simulink model "CR"  (R2020a)
settings: Solver=FixedStepAuto  StartTime=0.0  StopTime=0.02  FixedStep=1e-6  RelTol=1e-3
values from neighbouring files (symbols this model uses):
  A = 50    [injecktion.m]
  A_cyl = (pi*i_n/4)*d_noz^2    (= 4.31247208956e-07)    [injecktion.m]
  A_i = pi/4*d_i^2    (= 8.04247719319e-06)    [injecktion.m]
  A_n = (pi/4)*d_n^2    (= 6.93977817178e-05)    [injecktion.m]
  A_p = (pi/4)*d_p^2    (= 6.93977817178e-05)    [injecktion.m]
  A_pis = (pi/4)*d_p^2    (= 6.93977817178e-05)    [injecktion.m]
  A_s = (pi/4)*d_s^2    (= 3.63168110755e-05)    [injecktion.m]
  A_v = (pi/4)*d_c^2    (= 8.04247719319e-06)    [injecktion.m]
  angl = kamaz{1:720,1} - 180    [injecktion.m]
  angl_inj = [150 166.5 166.6 169.4 169.5 180.2 180.3 200]    [injecktion.m]
  B = -20    [injecktion.m]
  b_b = 0.2    [injecktion.m]
  b_n = 0.3    [injecktion.m]
  C_di = 0.85    [injecktion.m]
  Hv_max = 0.00052    [injecktion.m]
  K_n = 270000    [injecktion.m]
  K_v = 220000    [injecktion.m]
  L = 0.0002    [injecktion.m]
  m_a = 0.020    (= 0.02)    [injecktion.m]
  m_sum = 0.032    [injecktion.m]
  P_cyl = kamaz{1:720,2}    [injecktion.m]
  P_rail = 1800    [injecktion.m]
  P_t = 5    [injecktion.m]
  R = 1.1    [injecktion.m]
  rho = 832    [injecktion.m]
  V_inj = [0 0 60 60 40 40 0 0]    [injecktion.m]
libraries: simulink x1
settings Model: Creator=manun  LastModifiedBy=manun
settings SolverCC: AlgebraicLoopSolver=LineSearch

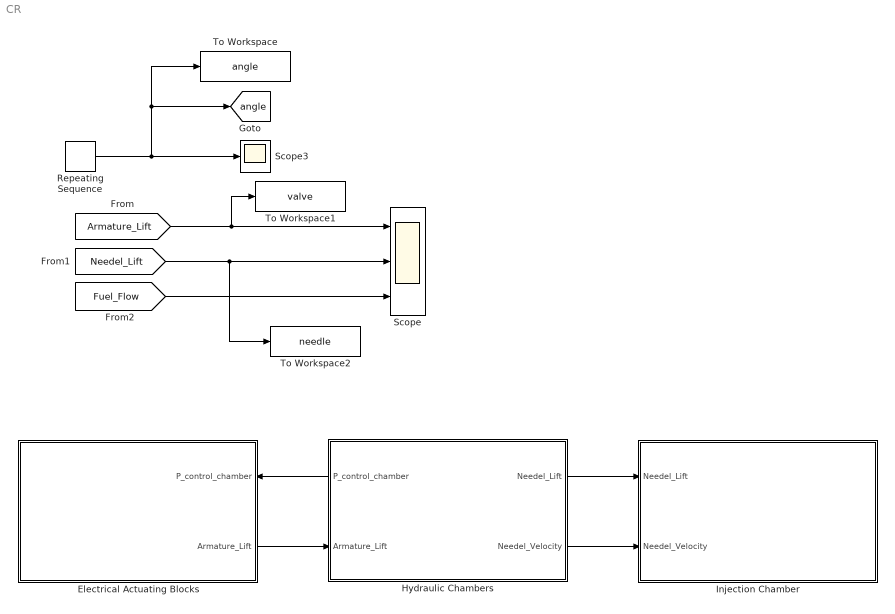
== system CR ==
  Electrical Actuating Blocks : Subsystem
      settings: PortSchema="{\"entries\":[{\"content\":{\"sides\":[{\"content\":{\"connectorIds\":[]},\"type\":\"ConnectorPlacement.EquallySpacedRectSide\",\"uuid\":\"3ba77c4c-b8ba-4d77-9d68-8710a2d773ab\"},{\"content\":{\"connectorIds\":[\"In1\",\"Out1\"],\"side\":\"RIGHT\"},\"type\":\"ConnectorPlacement.EquallySpacedRectSide\",\"uuid\":\"fd57f4f6-7259-4663-815b-091bcd4e1737\"},{\"content\":{\"connectorIds\":[],\"side\":\"TOP\"},\"type\":\"ConnectorPlacement.EquallySpacedRectSide\",\"uuid\":\"95c5c282-81a4-45f7-9203-cb060914cd9c\"}]},\"type\":\"ConnectorPlacement.EquallySpacedConnector\",\"uuid\":\"804a231b-9b03-46bc-815b-f5b483ae5845\"}],\"packageUris\":[\"http://schema.mathworks.com/mf0/Connector/19700101\"],\"version\":\"1.0\"}"
  Hydraulic Chambers : Subsystem
      settings: PortSchema="{\"entries\":[{\"content\":{\"sides\":[{\"content\":{\"connectorIds\":[\"Out3\",\"In1\"]},\"type\":\"ConnectorPlacement.EquallySpacedRectSide\",\"uuid\":\"e260e5f4-acfe-4da7-b401-bae8e315cc37\"},{\"content\":{\"connectorIds\":[\"Out1\",\"Out2\"],\"side\":\"RIGHT\"},\"type\":\"ConnectorPlacement.EquallySpacedRectSide\",\"uuid\":\"01019c56-b8d4-4519-8d57-ed1d2bc069d1\"},{\"content\":{\"connectorIds\":[],\"side\":\"TOP\"},\"type\":\"ConnectorPlacement.EquallySpacedRectSide\",\"uuid\":\"98af096b-7f3f-48cd-9514-e14eeceb55ee\"}]},\"type\":\"ConnectorPlacement.EquallySpacedConnector\",\"uuid\":\"efa95c2f-1e5f-488c-845f-cfa36b8d7348\"}],\"packageUris\":[\"http://schema.mathworks.com/mf0/Connector/19700101\"],\"version\":\"1.0\"}"
  Injection Chamber : Subsystem
  Repeating Sequence : simulink/Sources/Repeating Sequence  rep_seq_t=[0 0.0632]  rep_seq_y=[0 720]
  Scope : Scope  NumInputPorts=3
  Scope3 : Scope
  To Workspace : ToWorkspace  VariableName=angle  SampleTime=-1
  To Workspace1 : ToWorkspace  VariableName=valve  SaveFormat=Timeseries  SampleTime=-1
  To Workspace2 : ToWorkspace  VariableName=needle  SaveFormat=Timeseries  SampleTime=-1
  tag scope: angle=global
  wires:
  Repeating Sequence/1 -> To Workspace/1, [angle], Scope3/1
  Electrical Actuating Blocks/1(Armature_Lift) -> Hydraulic Chambers/1(Armature_Lift)
  Hydraulic Chambers/3(P_control_chamber) -> Electrical Actuating Blocks/1(P_control_chamber)
  Hydraulic Chambers/1(Needel_Lift) -> Injection Chamber/1(Needel_Lift)
  Hydraulic Chambers/2(Needel_Velocity) -> Injection Chamber/2(Needel_Velocity)
  [Armature_Lift] -> To Workspace1/1, Scope/1
  [Needel_Lift] -> To Workspace2/1, Scope/2
  [Fuel_Flow] -> Scope/3

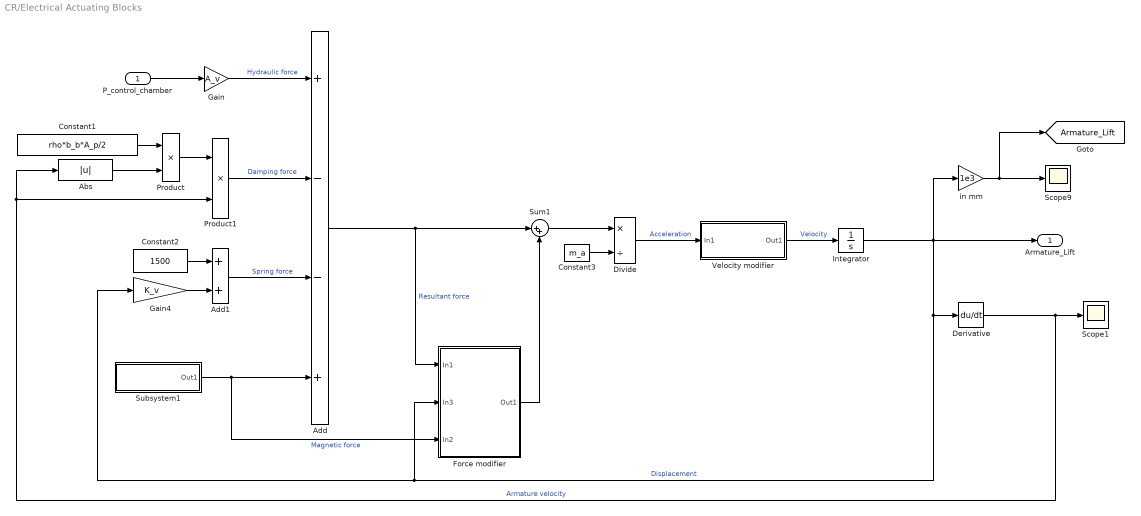
== system CR/Electrical Actuating Blocks ==
  P_control_chamber : Inport
  Abs : Abs
  Add : Sum  Inputs=+--+
  Add1 : Sum
  Constant1 : Constant  Value=rho*b_b*A_p/2
  Constant2 : Constant  Value=1500
  Constant3 : Constant  Value=m_a
  Derivative : Derivative
  Divide : Product  Inputs=*/
  Force modifier : Subsystem
  Gain : Gain  Gain=A_v
  Gain4 : Gain  Gain=K_v
  Integrator : Integrator  LimitOutput=on  UpperSaturationLimit=Hv_max  LowerSaturationLimit=0
  Product : Product
  Product1 : Product
  Scope1 : Scope
  Scope9 : Scope
  Subsystem1 : Subsystem
  Sum1 : Sum  Inputs=|++
  Velocity modifier : Subsystem
  in mm : Gain  Gain=1e3
  Armature_Lift : Outport
  tag scope: Armature_Lift=global
  wires:
  Integrator/1 -> Force modifier/2(In3), Gain4/1, Derivative/1, Armature_Lift/1, in mm/1  "Displacement"
  Constant3/1 -> Divide/2
  Gain4/1 -> Add1/2
  Sum1/1 -> Divide/1
  Add/1 -> Force modifier/1(In1), Sum1/1  "Resultant force"
  Abs/1 -> Product/2
  Velocity modifier/1(Out1) -> Integrator/1  "Velocity"
  P_control_chamber/1 -> Gain/1
  Product1/1 -> Add/2  "Damping force"
  Force modifier/1(Out1) -> Sum1/2
  Derivative/1 -> Scope1/1, Product1/2, Abs/1  "Armature velocity"
  Divide/1 -> Velocity modifier/1(In1)  "Acceleration"
  Product/1 -> Product1/1
  Constant2/1 -> Add1/1
  Subsystem1/1(Out1) -> Force modifier/3(In2), Add/4  "Magnetic force"
  Gain/1 -> Add/1  "Hydraulic force"
  Constant1/1 -> Product/1
  in mm/1 -> [Armature_Lift], Scope9/1
  Add1/1 -> Add/3  "Spring force"

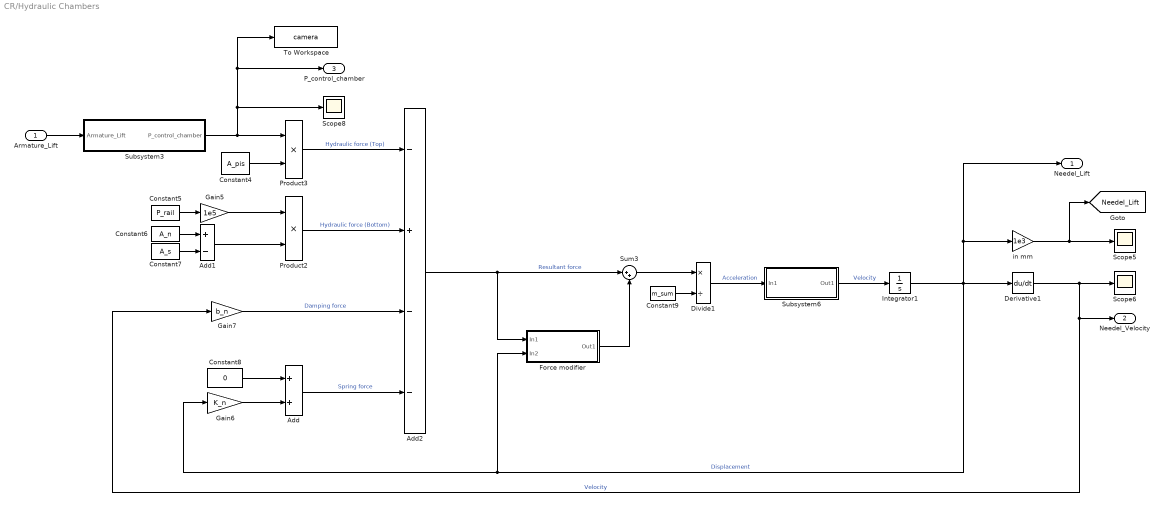
== system CR/Hydraulic Chambers ==
  Armature_Lift : Inport
  Add : Sum
  Add1 : Sum  Inputs=+-
  Add2 : Sum  Inputs=-+--
  Constant4 : Constant  Value=A_pis
  Constant5 : Constant  Value=P_rail
  Constant6 : Constant  Value=A_n
  Constant7 : Constant  Value=A_s
  Constant8 : Constant  Value=0
  Constant9 : Constant  Value=m_sum
  Derivative1 : Derivative
  Divide1 : Product  Inputs=*/
  Force modifier : Subsystem
  Gain5 : Gain  Gain=1e5
  Gain6 : Gain  Gain=K_n
  Gain7 : Gain  Gain=b_n
  Integrator1 : Integrator  LimitOutput=on  LowerSaturationLimit=0
  Product2 : Product
  Product3 : Product
  Scope5 : Scope
  Scope6 : Scope
  Scope8 : Scope
  Subsystem3 : Subsystem
  Subsystem6 : Subsystem
  Sum3 : Sum  Inputs=|++
  To Workspace : ToWorkspace  VariableName=camera  SaveFormat=Timeseries  SampleTime=-1
  in mm : Gain  Gain=1e3
  Needel_Lift : Outport
  Needel_Velocity : Outport  Port=2
  P_control_chamber : Outport  Port=3
  tag scope: Needel_Lift=global
  wires:
  in mm/1 -> [Needel_Lift], Scope5/1
  Derivative1/1 -> Gain7/1, Needel_Velocity/1, Scope6/1  "Velocity"
  Constant8/1 -> Add/1
  Force modifier/1(Out1) -> Sum3/2
  Integrator1/1 -> Gain6/1, Force modifier/2(In2), Needel_Lift/1, in mm/1, Derivative1/1  "Displacement"
  Subsystem6/1(Out1) -> Integrator1/1  "Velocity"
  Constant9/1 -> Divide1/2
  Product3/1 -> Add2/1  "Hydraulic force (Top)"
  Add/1 -> Add2/4  "Spring force"
  Gain7/1 -> Add2/3  "Damping force"
  Gain6/1 -> Add/2
  Sum3/1 -> Divide1/1
  Divide1/1 -> Subsystem6/1(In1)  "Acceleration"
  Constant5/1 -> Gain5/1
  Gain5/1 -> Product2/1
  Constant7/1 -> Add1/2
  Constant6/1 -> Add1/1
  Add2/1 -> Sum3/1, Force modifier/1(In1)  "Resultant force"
  Add1/1 -> Product2/2
  Constant4/1 -> Product3/2
  Product2/1 -> Add2/2  "Hydraulic force (Bottom)"
  Subsystem3/1(P_control_chamber) -> To Workspace/1, P_control_chamber/1, Scope8/1, Product3/1
  Armature_Lift/1 -> Subsystem3/1(Armature_Lift)

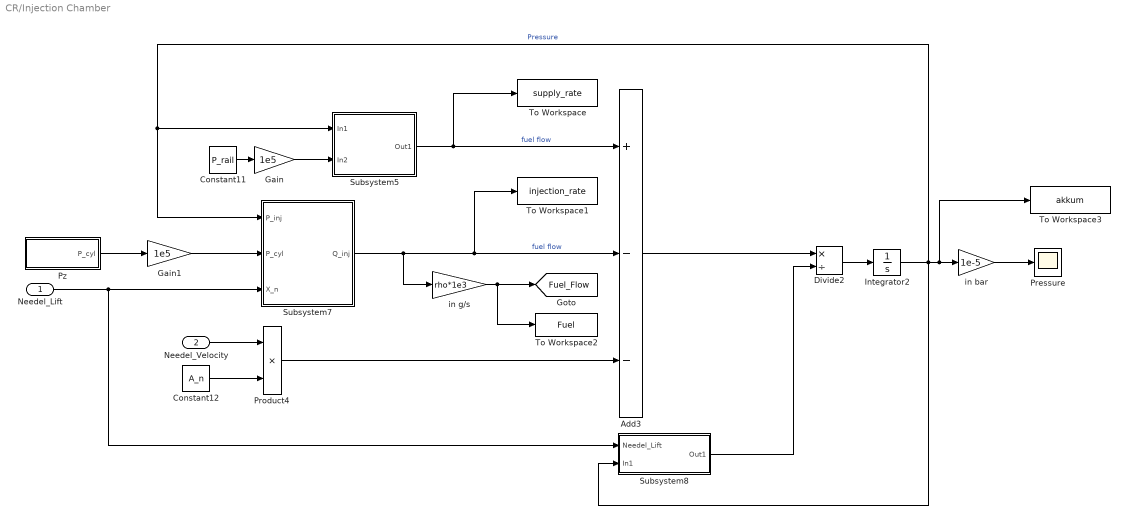
== system CR/Injection Chamber ==
  Needel_Lift : Inport
  Needel_Velocity : Inport  Port=2
  Add3 : Sum  Inputs=+--
  Constant11 : Constant  Value=P_rail
  Constant12 : Constant  Value=A_n
  Divide2 : Product  Inputs=*/
  Gain : Gain  Gain=1e5
  Gain1 : Gain  Gain=1e5
  Integrator2 : Integrator  InitialCondition=(P_rail)*1e5  LimitOutput=on  UpperSaturationLimit=(P_rail)*1e5  LowerSaturationLimit=1e5
  Pressure : Scope
  Product4 : Product
  Pz : Subsystem
  Subsystem5 : Subsystem
  Subsystem7 : Subsystem
  Subsystem8 : Subsystem
  To Workspace : ToWorkspace  VariableName=supply_rate  SaveFormat=Timeseries  SampleTime=-1
  To Workspace1 : ToWorkspace  VariableName=injection_rate  SaveFormat=Timeseries  SampleTime=-1
  To Workspace2 : ToWorkspace  VariableName=Fuel  SaveFormat=Timeseries  SampleTime=-1
      settings: Save2DSignal=2-D array (concatenate along first dimension)
  To Workspace3 : ToWorkspace  VariableName=akkum  SaveFormat=Timeseries  SampleTime=-1
  in bar : Gain  Gain=1e-5
  in g/s : Gain  Gain=rho*1e3
  tag scope: Fuel_Flow=global
  wires:
  Add3/1 -> Divide2/1
  Constant12/1 -> Product4/2
  Divide2/1 -> Integrator2/1
  Constant11/1 -> Gain/1
  Integrator2/1 -> Subsystem7/1(P_inj), Subsystem5/1(In1), Subsystem8/2(In1), To Workspace3/1, in bar/1  "Pressure"
  Pz/1(P_cyl) -> Gain1/1
  Subsystem5/1(Out1) -> To Workspace/1, Add3/1  "fuel flow"
  Subsystem7/1(Q_inj) -> in g/s/1, To Workspace1/1, Add3/2  "fuel flow"
  Gain/1 -> Subsystem5/2(In2)
  in g/s/1 -> [Fuel_Flow], To Workspace2/1
  Gain1/1 -> Subsystem7/2(P_cyl)
  Needel_Lift/1 -> Subsystem8/1(Needel_Lift), Subsystem7/3(X_n)
  Subsystem8/1(Out1) -> Divide2/2
  Needel_Velocity/1 -> Product4/1
  Product4/1 -> Add3/3
  in bar/1 -> Pressure/1

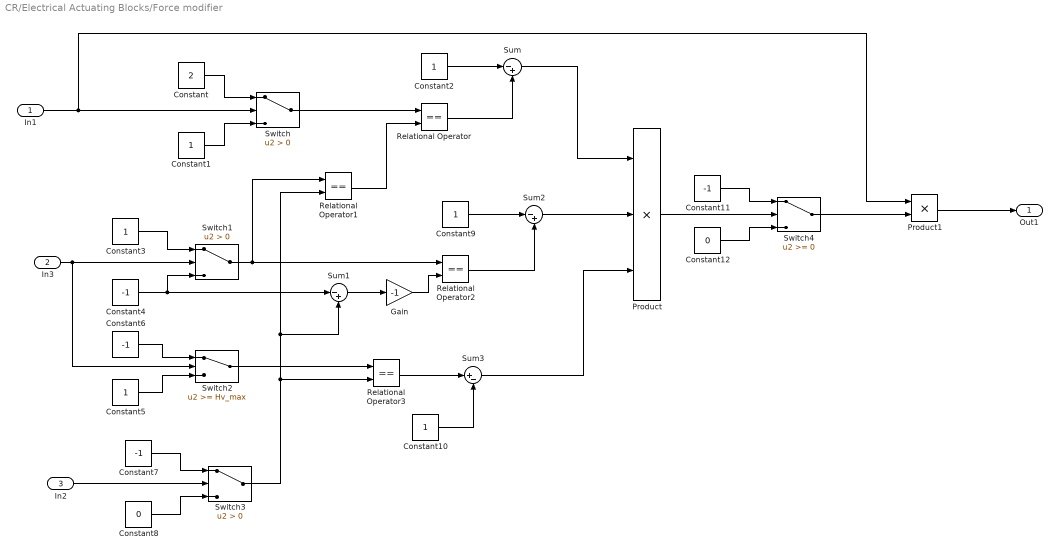
== system CR/Electrical Actuating Blocks/Force modifier ==
  In1 : Inport
  In3 : Inport  Port=2
  In2 : Inport  Port=3
  Constant : Constant  Value=2
  Constant{1..3,5,9..10} (6 alike) : Constant
  Constant{4,6..7,11} (4 alike) : Constant  Value=-1
  Constant12 : Constant  Value=0
  Constant8 : Constant  Value=0
  Gain : Gain  Gain=-1
  Product : Product  Inputs=3
  Product1 : Product
  Relational Operator{,1..3} (4 alike) : RelationalOperator  Operator===  OutDataTypeStr=boolean  RndMeth=Simplest
  Sum : Sum  Inputs=|-+
  Sum1 : Sum  Inputs=|-+
  Sum2 : Sum  Inputs=|-+
  Sum3 : Sum  Inputs=|+-
  Switch : Switch  Criteria=u2 > Threshold
  Switch1 : Switch  Criteria=u2 > Threshold
  Switch2 : Switch  Threshold=Hv_max
  Switch3 : Switch  Criteria=u2 > Threshold
  Switch4 : Switch
  Out1 : Outport
  wires:
  In1/1 -> Product1/1, Switch/2
  Constant/1 -> Switch/1
  Constant1/1 -> Switch/3
  Constant2/1 -> Sum/1
  Relational Operator/1 -> Sum/2
  Relational Operator1/1 -> Relational Operator/2
  Constant3/1 -> Switch1/1
  Constant4/1 -> Sum1/1, Switch1/3
  Switch1/1 -> Relational Operator1/1, Relational Operator2/1
  Switch3/1 -> Sum1/2, Relational Operator1/2, Relational Operator3/2
  In3/1 -> Switch2/2, Switch1/2
  Constant7/1 -> Switch3/1
  Constant8/1 -> Switch3/3
  In2/1 -> Switch3/2
  Switch2/1 -> Relational Operator3/1
  Gain/1 -> Relational Operator2/2
  Switch/1 -> Relational Operator/1
  Sum1/1 -> Gain/1
  Constant9/1 -> Sum2/1
  Relational Operator2/1 -> Sum2/2
  Sum2/1 -> Product/2
  Sum/1 -> Product/1
  Relational Operator3/1 -> Sum3/1
  Constant10/1 -> Sum3/2
  Sum3/1 -> Product/3
  Product/1 -> Switch4/2
  Constant12/1 -> Switch4/3
  Constant11/1 -> Switch4/1
  Switch4/1 -> Product1/2
  Product1/1 -> Out1/1
  Constant5/1 -> Switch2/3
  Constant6/1 -> Switch2/1

== system CR/Electrical Actuating Blocks/Subsystem1 ==
  Add : Sum
  Constant : Constant  Value=B
  Gain : Gain  Gain=A
  Subsystem : Subsystem
  Out1 : Outport
  wires:
  Gain/1 -> Add/1
  Add/1 -> Out1/1
  Constant/1 -> Add/2
  Subsystem/1(cur) -> Gain/1

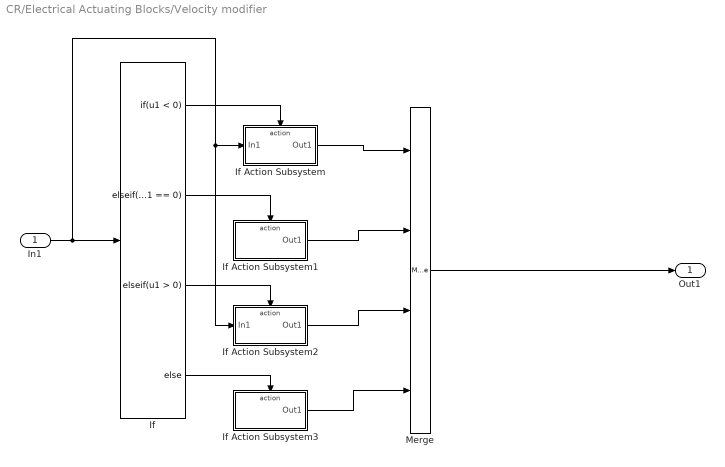
== system CR/Electrical Actuating Blocks/Velocity modifier ==
  In1 : Inport
  If : If  IfExpression=u1 < 0  ElseIfExpressions=u1 == 0, u1 > 0
  If Action Subsystem : Subsystem  TreatAsAtomicUnit=on
  If Action Subsystem1 : Subsystem  TreatAsAtomicUnit=on
  If Action Subsystem2 : Subsystem  TreatAsAtomicUnit=on
  If Action Subsystem3 : Subsystem  TreatAsAtomicUnit=on
  Merge : Merge  Inputs=4
  Out1 : Outport
  wires:
  In1/1 -> If Action Subsystem2/1(In1), If Action Subsystem/1(In1), If/1
  If/1 -> If Action Subsystem/Action
  If/2 -> If Action Subsystem1/Action
  If/3 -> If Action Subsystem2/Action
  If/4 -> If Action Subsystem3/Action
  If Action Subsystem/1(Out1) -> Merge/1
  If Action Subsystem1/1(Out1) -> Merge/2
  If Action Subsystem2/1(Out1) -> Merge/3
  If Action Subsystem3/1(Out1) -> Merge/4
  Merge/1 -> Out1/1

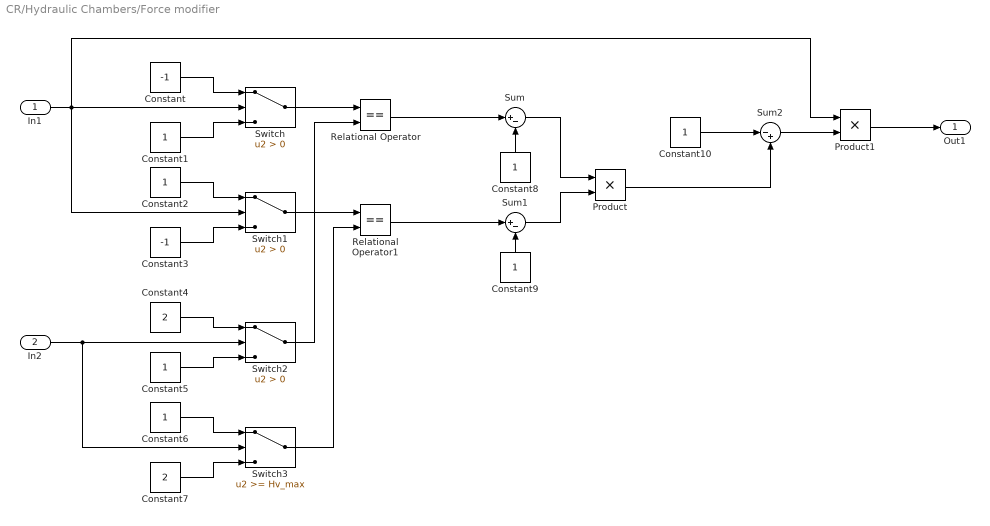
== system CR/Hydraulic Chambers/Force modifier ==
  In1 : Inport
  In2 : Inport  Port=2
  Constant : Constant  Value=-1
  Constant{1..2,5..6,8..10} (7 alike) : Constant
  Constant3 : Constant  Value=-1
  Constant4 : Constant  Value=2
  Constant7 : Constant  Value=2
  Product : Product
  Product1 : Product
  Relational Operator : RelationalOperator  Operator===  OutDataTypeStr=boolean  RndMeth=Simplest
  Relational Operator1 : RelationalOperator  Operator===  OutDataTypeStr=boolean  RndMeth=Simplest
  Sum : Sum  Inputs=|+-
  Sum1 : Sum  Inputs=|+-
  Sum2 : Sum  Inputs=|-+
  Switch : Switch  Criteria=u2 > Threshold
  Switch1 : Switch  Criteria=u2 > Threshold
  Switch2 : Switch  Criteria=u2 > Threshold
  Switch3 : Switch  Threshold=Hv_max
  Out1 : Outport
  wires:
  Constant/1 -> Switch/1
  Constant1/1 -> Switch/3
  Switch/1 -> Relational Operator/1
  In1/1 -> Product1/1, Switch1/2, Switch/2
  Constant2/1 -> Switch1/1
  Constant3/1 -> Switch1/3
  Switch1/1 -> Relational Operator1/1
  Switch3/1 -> Relational Operator1/2
  Constant6/1 -> Switch3/1
  Constant7/1 -> Switch3/3
  Switch2/1 -> Relational Operator/2
  In2/1 -> Switch3/2, Switch2/2
  Relational Operator/1 -> Sum/1
  Relational Operator1/1 -> Sum1/1
  Constant8/1 -> Sum/2
  Constant9/1 -> Sum1/2
  Sum/1 -> Product/1
  Sum1/1 -> Product/2
  Constant10/1 -> Sum2/1
  Product1/1 -> Out1/1
  Product/1 -> Sum2/2
  Sum2/1 -> Product1/2
  Constant4/1 -> Switch2/1
  Constant5/1 -> Switch2/3

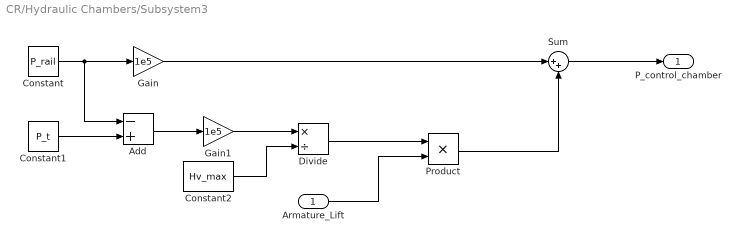
== system CR/Hydraulic Chambers/Subsystem3 ==
  Armature_Lift : Inport
  Add : Sum  Inputs=-+
  Constant : Constant  Value=P_rail
  Constant1 : Constant  Value=P_t
  Constant2 : Constant  Value=Hv_max
  Divide : Product  Inputs=*/
  Gain : Gain  Gain=1e5
  Gain1 : Gain  Gain=1e5
  Product : Product
  Sum : Sum  Inputs=|++
  P_control_chamber : Outport
  wires:
  Constant/1 -> Add/1, Gain/1
  Constant1/1 -> Add/2
  Add/1 -> Gain1/1
  Gain1/1 -> Divide/1
  Constant2/1 -> Divide/2
  Divide/1 -> Product/1
  Armature_Lift/1 -> Product/2
  Product/1 -> Sum/2
  Gain/1 -> Sum/1
  Sum/1 -> P_control_chamber/1

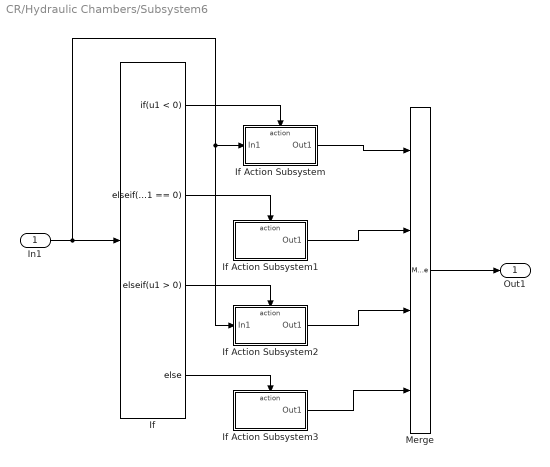
== system CR/Hydraulic Chambers/Subsystem6 ==
  In1 : Inport
  If : If  IfExpression=u1 < 0  ElseIfExpressions=u1 == 0, u1 > 0
  If Action Subsystem : Subsystem  TreatAsAtomicUnit=on
  If Action Subsystem1 : Subsystem  TreatAsAtomicUnit=on
  If Action Subsystem2 : Subsystem  TreatAsAtomicUnit=on
  If Action Subsystem3 : Subsystem  TreatAsAtomicUnit=on
  Merge : Merge  Inputs=4
  Out1 : Outport
  wires:
  In1/1 -> If Action Subsystem2/1(In1), If Action Subsystem/1(In1), If/1
  Merge/1 -> Out1/1
  If/1 -> If Action Subsystem/Action
  If/2 -> If Action Subsystem1/Action
  If/3 -> If Action Subsystem2/Action
  If/4 -> If Action Subsystem3/Action
  If Action Subsystem/1(Out1) -> Merge/1
  If Action Subsystem1/1(Out1) -> Merge/2
  If Action Subsystem2/1(Out1) -> Merge/3
  If Action Subsystem3/1(Out1) -> Merge/4

== system CR/Injection Chamber/Pz ==
  1-D Lookup Table : Lookup_n-D  NumberOfTableDimensions=1  BreakpointsForDimension1=angl  Table=P_cyl  InternalRulePriority=Speed  RndMeth=Simplest  InputSameDT=on
  P_cyl : Outport
  wires:
  [angle] -> 1-D Lookup Table/1
  1-D Lookup Table/1 -> P_cyl/1

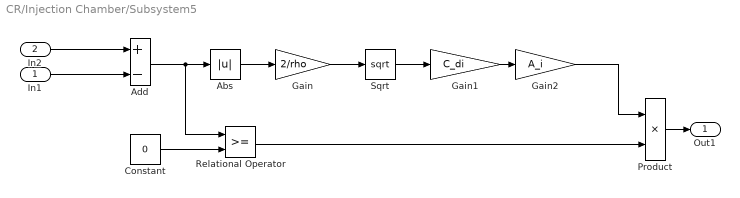
== system CR/Injection Chamber/Subsystem5 ==
  In1 : Inport
  In2 : Inport  Port=2
  Abs : Abs
  Add : Sum  Inputs=+-
  Constant : Constant  Value=0
  Gain : Gain  Gain=2/rho
  Gain1 : Gain  Gain=C_di
  Gain2 : Gain  Gain=A_i
  Product : Product
  Relational Operator : RelationalOperator  OutDataTypeStr=boolean  RndMeth=Simplest
  Sqrt : Sqrt  SaturateOnIntegerOverflow=on
  Out1 : Outport
  wires:
  Gain1/1 -> Gain2/1
  Add/1 -> Relational Operator/1, Abs/1
  Sqrt/1 -> Gain1/1
  Abs/1 -> Gain/1
  Gain/1 -> Sqrt/1
  In1/1 -> Add/2
  In2/1 -> Add/1
  Product/1 -> Out1/1
  Gain2/1 -> Product/1
  Constant/1 -> Relational Operator/2
  Relational Operator/1 -> Product/2

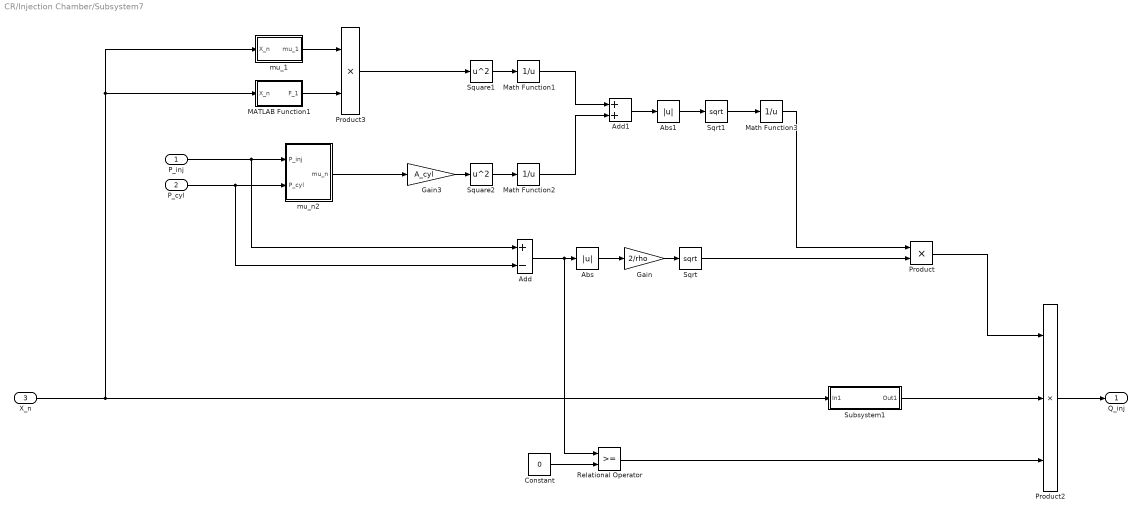
== system CR/Injection Chamber/Subsystem7 ==
  P_inj : Inport
  P_cyl : Inport  Port=2
  X_n : Inport  Port=3
  Abs : Abs
  Abs1 : Abs
  Add : Sum  Inputs=+-
  Add1 : Sum
  Constant : Constant  Value=0
  Gain : Gain  Gain=2/rho
  Gain3 : Gain  Gain=A_cyl
  MATLAB Function1 : MATLAB Function  TreatAsAtomicUnit=on
  Math Function1 : Math  Operator=reciprocal  SignedPower=on  RndMeth=Zero  SaturateOnIntegerOverflow=on
  Math Function2 : Math  Operator=reciprocal  SignedPower=on  RndMeth=Zero  SaturateOnIntegerOverflow=on
  Math Function3 : Math  Operator=reciprocal  SignedPower=on  RndMeth=Zero  SaturateOnIntegerOverflow=on
  Product : Product
  Product2 : Product  Inputs=3
  Product3 : Product
  Relational Operator : RelationalOperator  OutDataTypeStr=boolean  RndMeth=Simplest
  Sqrt : Sqrt  SaturateOnIntegerOverflow=on
  Sqrt1 : Sqrt  SaturateOnIntegerOverflow=on
  Square1 : Math  Operator=square  SaturateOnIntegerOverflow=on
  Square2 : Math  Operator=square  SaturateOnIntegerOverflow=on
  Subsystem1 : Subsystem
  mu_1 : MATLAB Function  TreatAsAtomicUnit=on
  mu_n2 : MATLAB Function  TreatAsAtomicUnit=on
  Q_inj : Outport
  wires:
  Subsystem1/1(Out1) -> Product2/2
  Product2/1 -> Q_inj/1
  mu_n2/1(mu_n) -> Gain3/1
  mu_1/1(mu_1) -> Product3/1
  Product3/1 -> Square1/1
  Square1/1 -> Math Function1/1
  MATLAB Function1/1(F_1) -> Product3/2
  Product/1 -> Product2/1
  P_cyl/1 -> mu_n2/2(P_cyl), Add/2
  P_inj/1 -> Add/1, mu_n2/1(P_inj)
  X_n/1 -> Subsystem1/1(In1), mu_1/1(X_n), MATLAB Function1/1(X_n)
  Gain/1 -> Sqrt/1
  Abs/1 -> Gain/1
  Relational Operator/1 -> Product2/3
  Constant/1 -> Relational Operator/2
  Add/1 -> Relational Operator/1, Abs/1
  Square2/1 -> Math Function2/1
  Gain3/1 -> Square2/1
  Math Function1/1 -> Add1/1
  Math Function2/1 -> Add1/2
  Add1/1 -> Abs1/1
  Abs1/1 -> Sqrt1/1
  Sqrt1/1 -> Math Function3/1
  Math Function3/1 -> Product/1
  Sqrt/1 -> Product/2

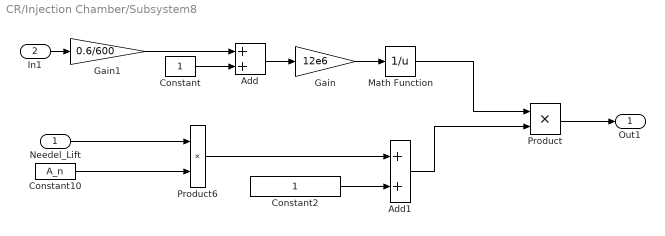
== system CR/Injection Chamber/Subsystem8 ==
  Needel_Lift : Inport
  In1 : Inport  Port=2
  Add : Sum
  Add1 : Sum
  Constant : Constant
  Constant10 : Constant  Value=A_n
  Constant2 : Constant
  Gain : Gain  Gain=12e6
  Gain1 : Gain  Gain=0.6/600
  Math Function : Math  Operator=reciprocal  SaturateOnIntegerOverflow=on
  Product : Product
  Product6 : Product
  Out1 : Outport
  wires:
  Constant/1 -> Add/2
  Add/1 -> Gain/1
  Gain1/1 -> Add/1
  Constant2/1 -> Add1/2
  Product/1 -> Out1/1
  Constant10/1 -> Product6/2
  Product6/1 -> Add1/1
  Add1/1 -> Product/2
  Needel_Lift/1 -> Product6/1
  Gain/1 -> Math Function/1
  In1/1 -> Gain1/1
  Math Function/1 -> Product/1

== system CR/Electrical Actuating Blocks/Subsystem1/Subsystem ==
  Add : Sum  Inputs=+-
  Derivative : Derivative
  Gain : Gain  Gain=1/R
  Gain1 : Gain  Gain=L
  To Workspace : ToWorkspace  VariableName=V  SaveFormat=Timeseries  SampleTime=-1
  To Workspace1 : ToWorkspace  VariableName=I  SaveFormat=Timeseries  SampleTime=-1
  V : Subsystem
  cur : Outport
  wires:
  Add/1 -> Gain/1
  Derivative/1 -> Gain1/1
  Gain1/1 -> Add/2
  V/1(Out1) -> To Workspace/1, Add/1
  Gain/1 -> Derivative/1, To Workspace1/1, cur/1

== system CR/Electrical Actuating Blocks/Velocity modifier/If Action Subsystem ==
  In1 : Inport
  Action Port : ActionPort  ActionPortLabel=if(u1 < 0)
  Integrator : Integrator
  Out1 : Outport
  wires:
  In1/1 -> Integrator/1
  Integrator/1 -> Out1/1

== system CR/Electrical Actuating Blocks/Velocity modifier/If Action Subsystem1 ==
  Action Port : ActionPort  ActionPortLabel=elseif(u1 == 0)
  Constant : Constant  Value=0
  Out1 : Outport
  wires:
  Constant/1 -> Out1/1

== system CR/Electrical Actuating Blocks/Velocity modifier/If Action Subsystem2 ==
  In1 : Inport
  Action Port : ActionPort  ActionPortLabel=elseif( u1 > 0)
  Integrator : Integrator
  Out1 : Outport
  wires:
  In1/1 -> Integrator/1
  Integrator/1 -> Out1/1

== system CR/Electrical Actuating Blocks/Velocity modifier/If Action Subsystem3 ==
  Action Port : ActionPort  ActionPortLabel=else
  Constant : Constant  Value=0
  Out1 : Outport
  wires:
  Constant/1 -> Out1/1

== system CR/Hydraulic Chambers/Subsystem6/If Action Subsystem ==
  In1 : Inport
  Action Port : ActionPort  ActionPortLabel=if(u1 < 0)
  Integrator : Integrator
  Out1 : Outport
  wires:
  In1/1 -> Integrator/1
  Integrator/1 -> Out1/1

== system CR/Hydraulic Chambers/Subsystem6/If Action Subsystem1 ==
  Action Port : ActionPort  ActionPortLabel=elseif(u1 == 0)
  Constant : Constant  Value=0
  Out1 : Outport
  wires:
  Constant/1 -> Out1/1

== system CR/Hydraulic Chambers/Subsystem6/If Action Subsystem2 ==
  In1 : Inport
  Action Port : ActionPort  ActionPortLabel=elseif( u1 > 0)
  Integrator : Integrator
  Out1 : Outport
  wires:
  In1/1 -> Integrator/1
  Integrator/1 -> Out1/1

== system CR/Hydraulic Chambers/Subsystem6/If Action Subsystem3 ==
  Action Port : ActionPort  ActionPortLabel=else
  Constant : Constant  Value=0
  Out1 : Outport
  wires:
  Constant/1 -> Out1/1

== system CR/Injection Chamber/Subsystem7/Subsystem1 ==
  In1 : Inport
  Constant : Constant  Value=0
  Constant2 : Constant
  Switch : Switch  Criteria=u2 > Threshold
  Out1 : Outport
  wires:
  In1/1 -> Switch/2
  Switch/1 -> Out1/1
  Constant/1 -> Switch/3
  Constant2/1 -> Switch/1

== system CR/Electrical Actuating Blocks/Subsystem1/Subsystem/V ==
  1-D Lookup Table : Lookup_n-D  NumberOfTableDimensions=1  BreakpointsForDimension1=angl_inj  Table=V_inj  InternalRulePriority=Speed  RndMeth=Simplest  InputSameDT=on
  Out1 : Outport
  wires:
  1-D Lookup Table/1 -> Out1/1
  [angle] -> 1-D Lookup Table/1

== matlab function CR/Injection Chamber/Subsystem7/MATLAB Function1 ==
  data: X_n input; F_1 output
function F_1 = fcn(X_n)

F_1 = X_n*sin(60*pi/180)*pi*((0.0028)+X_n*sin(60*pi/180)*cos(60*pi/180));

end

== matlab function CR/Injection Chamber/Subsystem7/mu_n2 ==
  data: P_inj input; mu_n output; P_cyl input
function mu_n = fcn(P_inj, P_cyl)

K = (P_inj - P_cyl)/P_cyl;
mu_atm = 0.4;

if K > 1.5
    mu_n = mu_atm + 4.6/((K+6)^1.7);
else
    mu_n = mu_atm + 0.15;
end
end

== matlab function CR/Injection Chamber/Subsystem7/mu_1 ==
  data: X_n input; mu_1 output
function mu_1 = fcn(X_n)

mu_1 = 1/(2.096-4.229*(10^6)*X_n^2);
